simulink model "modeloMalhaFechada"  (R2021a)
settings: Solver=VariableStepAuto  StartTime=0.0  StopTime=1000  RelTol=1e-3
values from neighbouring files (symbols this model uses):
  ganhoFF = tfVentiladorResfriamento/tfAquecedorAquecimento    [calculoControlador.m]
libraries: cstblocks x4
settings Model: Creator=pedroian  LastModifiedBy=pedroian

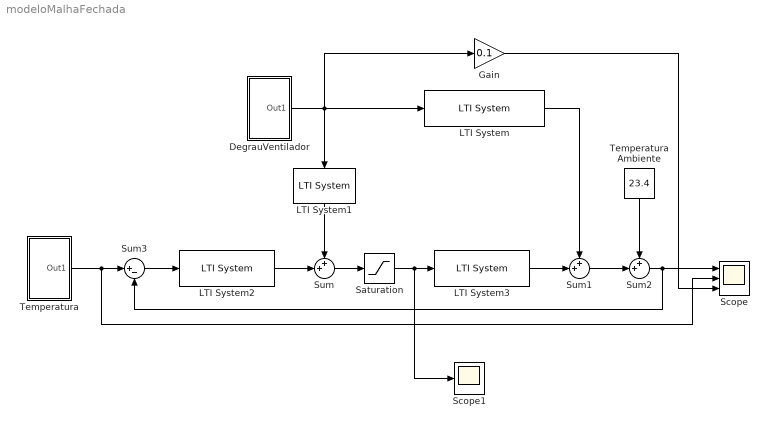
== system modeloMalhaFechada ==
  DegrauVentilador : Subsystem
  Gain : Gain  Gain=0.1
  LTI System : cstblocks/LTI System  sys=tfVentiladorResfriamento  IC=[]
  LTI System1 : cstblocks/LTI System  sys=-ganhoFF  IC=[]
  LTI System2 : cstblocks/LTI System  sys=GControladorAA  IC=[]
  LTI System3 : cstblocks/LTI System  sys=tfAquecedorAquecimento  IC=[]
  Saturation : Saturate  UpperLimit=200  LowerLimit=0  ZeroCross=off
  Scope : Scope  NumInputPorts=3
  Scope1 : Scope
  Sum : Sum  Inputs=++|
  Sum1 : Sum  Inputs=++|
  Sum2 : Sum  Inputs=++|
  Sum3 : Sum  Inputs=|+-
  Temperatura : Subsystem
  Temperatura Ambiente : Constant  Value=23.4
  wires:
  DegrauVentilador/1(Out1) -> Gain/1, LTI System1/1, LTI System/1
  Temperatura/1(Out1) -> Sum3/1, Scope/2
  LTI System2/1 -> Sum/2
  LTI System3/1 -> Sum1/2
  Temperatura Ambiente/1 -> Sum2/1
  Sum1/1 -> Sum2/2
  Sum2/1 -> Sum3/2, Scope/1
  Sum3/1 -> LTI System2/1
  LTI System1/1 -> Sum/1
  LTI System/1 -> Sum1/1
  Gain/1 -> Scope/3
  Sum/1 -> Saturation/1
  Saturation/1 -> Scope1/1, LTI System3/1

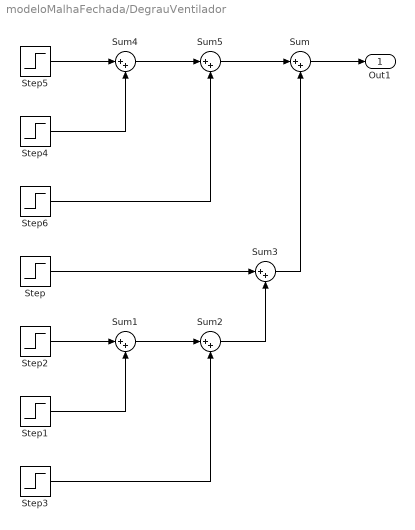
== system modeloMalhaFechada/DegrauVentilador ==
  Step : Step  Time=1200  After=-1000  SampleTime=0
  Step1 : Step  Time=1716  After=-500  SampleTime=0
  Step2 : Step  Time=1448  After=500  SampleTime=0
  Step3 : Step  Time=1997  After=1000  SampleTime=0
  Step4 : Step  Time=716  After=-500  SampleTime=0
  Step5 : Step  Time=448  After=500  SampleTime=0
  Step6 : Step  Time=997  After=1000  SampleTime=0
  Sum{,1..5} (6 alike) : Sum  Inputs=|++
  Out1 : Outport
  wires:
  Sum4/1 -> Sum5/1
  Step6/1 -> Sum5/2
  Step4/1 -> Sum4/2
  Step5/1 -> Sum4/1
  Step1/1 -> Sum1/2
  Step3/1 -> Sum2/2
  Sum1/1 -> Sum2/1
  Step2/1 -> Sum1/1
  Sum5/1 -> Sum/1
  Sum/1 -> Out1/1
  Sum2/1 -> Sum3/2
  Step/1 -> Sum3/1
  Sum3/1 -> Sum/2

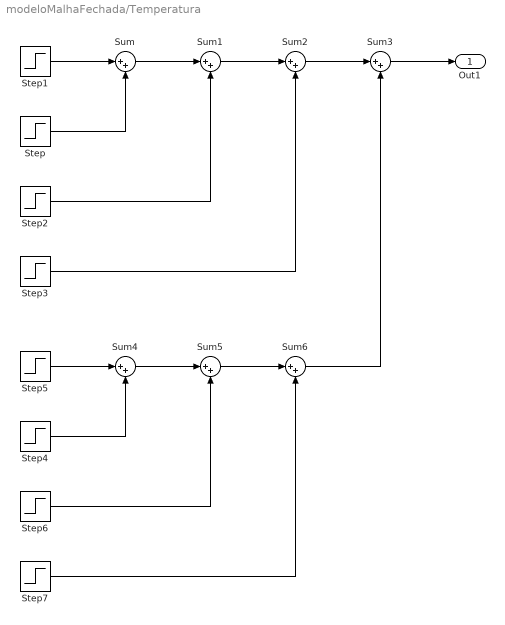
== system modeloMalhaFechada/Temperatura ==
  Step : Step  Time=399  After=25  SampleTime=0
  Step1 : Step  Time=84  After=25  SampleTime=0
  Step2 : Step  Time=844  After=25  SampleTime=0
  Step3 : Step  Time=1404  After=25  SampleTime=0
  Step4 : Step  Time=2225  After=-25  SampleTime=0
  Step5 : Step  Time=1632  After=-25  SampleTime=0
  Step6 : Step  Time=2874  After=-25  SampleTime=0
  Step7 : Step  Time=3545  After=-25  SampleTime=0
  Sum{,1..6} (7 alike) : Sum  Inputs=|++
  Out1 : Outport
  wires:
  Step2/1 -> Sum1/2
  Sum/1 -> Sum1/1
  Step/1 -> Sum/2
  Sum1/1 -> Sum2/1
  Step1/1 -> Sum/1
  Step3/1 -> Sum2/2
  Sum6/1 -> Sum3/2
  Step4/1 -> Sum4/2
  Step6/1 -> Sum5/2
  Step5/1 -> Sum4/1
  Step7/1 -> Sum6/2
  Sum4/1 -> Sum5/1
  Sum5/1 -> Sum6/1
  Sum2/1 -> Sum3/1
  Sum3/1 -> Out1/1
